simulink model "vehicle_dynamics_blockset_simulation"  (R2020b)
settings: Solver=VariableStepAuto  StartTime=0.0  StopTime=10.0  RelTol=1e-3
values from neighbouring files (symbols this model uses):
  CONST =     [ParamsFull.mat]
  VEHICLE =     [ParamsFull.mat]
undefined symbols (not defined in the file or in its folder): InertFrm, VEH
libraries: sharedtransform x6, sim3dlib x4, vehdynlibtirecommon x4, autolibutils x4, autolibshared x3, vehdynlibtire x2, vehdynlibviscommon x2, vehdynlibsteering x1, simulink x1, sim3dautolib x1
(part 1 of 4)
settings Model: Creator=josip  LastModifiedBy=josip
settings DataIOCC: ReturnWorkspaceOutputs=off
settings DebuggingCC: ArithmeticOperatorsInVariantConditions=warning
settings HardwareCC: ProdBitPerLong=64  ProdHWDeviceType=AMD->x86-64 (Linux 64)
settings SFSimCC: CustomCodeUndefinedFunction=UseInterfaceOnly

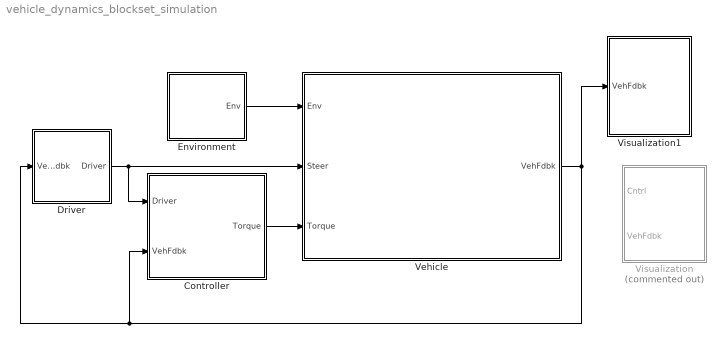
== system vehicle_dynamics_blockset_simulation ==
  Controller : Subsystem
      mask Display: image('images/SystemControllers.png')
  Driver : Subsystem  VariantControl=0
      mask Display: image('images/LongitudinalDriver.png');
  Environment : Subsystem
      mask Display: disp('Environment')
  Vehicle : Subsystem
      mask Display: image('images/PassengerVehicle.png')
  Visualization : Subsystem  Commented=on
      mask Display: disp('Visualization')
  Visualization1 : Subsystem
      mask Display: disp('Visualization')
  wires:
  Environment/1(Env) -> Vehicle/1(Env)
  Driver/1(Driver) -> Controller/1(Driver), Vehicle/2(Steer)
  Vehicle/1(VehFdbk) -> Visualization1/1(VehFdbk), Controller/2(VehFdbk), Driver/1(VehFdbk)
  Controller/1(Torque) -> Vehicle/3(Torque)

== system vehicle_dynamics_blockset_simulation/Controller ==
  Driver : Inport
  VehFdbk : Inport  Port=2
  Constant : Constant  Value=50*ones(4,1)
  Terminator : Terminator
  Terminator1 : Terminator
  Torque : Outport  VectorParamsAs1DForOutWhenUnconnected=off
  wires:
  Driver/1 -> Terminator/1
  VehFdbk/1 -> Terminator1/1
  Constant/1 -> Torque/1

== system vehicle_dynamics_blockset_simulation/Driver ==
  VehFdbk : Inport
  Brake : Constant  Value=0
  Bus Creator1 : BusCreator  Inputs=3
  Bus Selector : BusSelector  Commented=on  OutputSignals=BdyFrm.Cg.Vel.xdot
  Constant : Constant  Commented=on  Value=10
  Dead Zone : DeadZone  Commented=on  LowerValue=-.1  UpperValue=.1  SaturateOnIntegerOverflow=on
  Gas : Constant  Value=0.5
  Ground : Ground  Commented=on
  Longitudinal Driver : autolibshared/Longitudinal Driver  Commented=on  extAccelOvr=off  extDecelOvr=off  extAccelHld=off  extDecelHld=off  extAccelZero=off  extDecelZero=off  cntrlType=PI  shftType=None  velUnits=m/s  gearOut=off  Kp=10  Ki=5  Kff=.1  Kg=0  VehVelVec=[0 100]  KffVec=[.1 .1]  KpVec=[10 10]  KiVec=[5 5]  KgVec=[0 0]  m=1500  Kpt=3000  tau=.1  L=2  aR=200  bR=2.5  cR=.5  g=9.81  vnom=10  Kaw=0  tauerr=0  tauPt=2  GearInit=0  tShift=.1  pdlVec=[0.1 0.4 0.5 0.9]  upShftTbl=[-1 12.9375 26.4375 39.9375 51.18749999999999 62.4375 72.84375 83.25;-1 16.3125 29.8125 43.3125 54.5624 65.8125 76.78125 87.75;-1 19.6875 33.1875 46.68749999999999 57.9375 69.1875 80.71875 92.25;-1 33 52.5 77.25 100.5 138.75 161.875 185]  dwnShftTbl=[1 9.5625 23.0625 36.5625 47.8125 59.0625 68.90625 78.75;1 12.9375 26.4375 39.9375 51.18749999999999 62.4375 72.84375 83.25;1 16.3125 29.8125 43.3125 54.562499 65.8125 76.78125 87.75;1 19.6875 33.1875 46.68749999999999 57.9375 69.1875 80.71875 92.25]  tClutch=.5  tRev=.5  tPark=120  aMode=2  UpGearVec="[0  1  2  3  4  5  6  7]"  DownGearVec="[1  2  3  4  5  6  7  8]"
      settings: SourceProductBaseCode=PW,MT,UV,VE,VP
  Steer : Constant  Value=deg2rad(45)
  Terminator : Terminator
  Terminator1 : Terminator  Commented=on
  Terminator2 : Terminator  Commented=on
  Terminator3 : Terminator  Commented=on
  Driver : Outport  VectorParamsAs1DForOutWhenUnconnected=off
  wires:
  Longitudinal Driver/3 -> Terminator2/1  "Brake"
  Ground/1 -> Longitudinal Driver/3
  Longitudinal Driver/2 -> Terminator1/1  "Accel"
  Bus Creator1/1 -> Driver/1
  Longitudinal Driver/1 -> Terminator3/1
  Bus Selector/1 -> Dead Zone/1  "<xdot>"
  Dead Zone/1 -> Longitudinal Driver/2
  Constant/1 -> Longitudinal Driver/1
  Steer/1 -> Bus Creator1/1  "steer"
  Gas/1 -> Bus Creator1/2  "gas"
  Brake/1 -> Bus Creator1/3  "brake"
  VehFdbk/1 -> Terminator/1

== system vehicle_dynamics_blockset_simulation/Environment ==
  Bus Creator1 : BusCreator  Inputs=2
  Constant3 : Constant  Value=0
  Constant4 : Constant  Value=0
  Constant5 : Constant  Value=0
  Friction : Constant  Value=ones(4,1).*1.0
  Ground Feedback : Subsystem  Variant=on  VariantControlMode=label  LabelModeActiveChoice=0
  Vector Concatenate : Concatenate  NumInputs=3
  Env : Outport  VectorParamsAs1DForOutWhenUnconnected=off
  wires:
  Constant5/1 -> Vector Concatenate/3  "Z"
  Vector Concatenate/1 -> Bus Creator1/1  "Wind"
  Constant3/1 -> Vector Concatenate/1  "X"
  Constant4/1 -> Vector Concatenate/2  "Y"
  Ground Feedback/1(Ground) -> Bus Creator1/2  "Gnd"
  Bus Creator1/1 -> Env/1
  Friction/1 -> Ground Feedback/1(Friction)

== system vehicle_dynamics_blockset_simulation/Vehicle ==
  Env : Inport
  Steer : Inport  Port=2
  Torque : Inport  Port=3
  Bus Selector1 : BusSelector  OutputSignals=Gnd.z.G_FL_z,Gnd.z.G_FR_z,Gnd.z.G_RL_z,Gnd.z.G_RR_z
  Bus Selector2 : BusSelector  OutputSignals=Wind
  Bus Selector3 : BusSelector  OutputSignals=Gnd.mu.mu_FL,Gnd.mu.mu_FR,Gnd.mu.mu_RL,Gnd.mu.mu_RR
  Bus Selector4 : BusSelector  OutputSignals=steer
  Constant : Constant  Value=zeros(4,1)
  PassVeh7DOF : ModelReference  Commented=on  ModelNameDialog=PassVeh7DOF  SimulationMode=Normal  VariantControl=1  ModelReferenceVersion=2.89
  Steering : Subsystem
  Terminator : Terminator
  Vector Concatenate : Concatenate  NumInputs=4
  Vector Concatenate1 : Concatenate  NumInputs=4
  Vehicle : Subsystem
  Wheels and tires : Subsystem  Commented=on
  VehFdbk : Outport  VectorParamsAs1DForOutWhenUnconnected=off
  wires:
  Steer/1 -> Bus Selector4/1
  Steering/1(WhlAng) -> Vehicle/4(WhlAng)
  Torque/1 -> Vehicle/1(AxlTrq)
  Constant/1 -> Vehicle/2(BrkPrs)
  Vehicle/1(Veh) -> VehFdbk/1
  Bus Selector3/1 -> Vector Concatenate/1  "<mu_FL>"
  Bus Selector1/2 -> Vector Concatenate1/2  "<G_FR_z>"
  Vector Concatenate1/1 -> Vehicle/5(Ground)
  Vector Concatenate/1 -> Vehicle/6(Friction)
  Bus Selector1/1 -> Vector Concatenate1/1  "<G_FL_z>"
  Bus Selector3/4 -> Vector Concatenate/4  "<mu_RR>"
  Bus Selector3/2 -> Vector Concatenate/2  "<mu_FR>"
  Bus Selector3/3 -> Vector Concatenate/3  "<mu_RL>"
  Bus Selector1/4 -> Vector Concatenate1/4  "<G_RR_z>"
  Bus Selector1/3 -> Vector Concatenate1/3  "<G_RL_z>"
  Bus Selector2/1 -> Vehicle/3(WindXYZ)  "<Wind>"
  Env/1 -> Bus Selector3/1, Bus Selector1/1, Bus Selector2/1
  Vehicle/2(Wheels) -> Terminator/1
  Bus Selector4/1 -> Steering/1(Steer)  "<steer>"

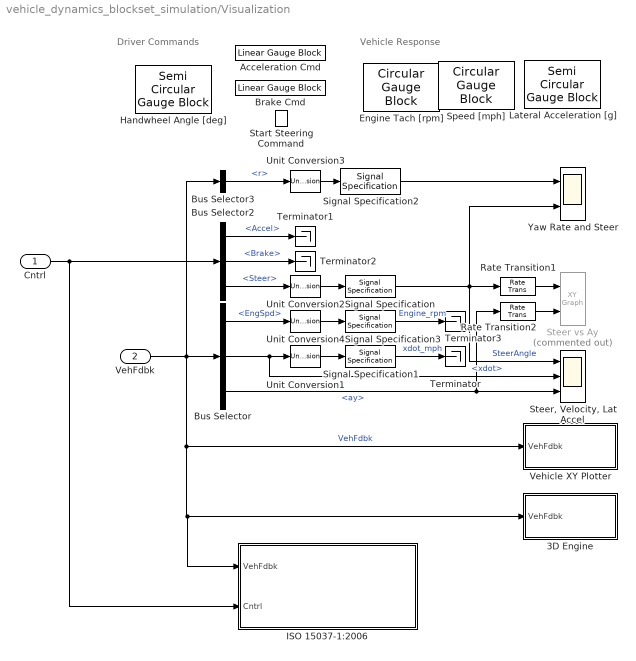
== system vehicle_dynamics_blockset_simulation/Visualization ==
  note: Driver Commands
  note: Vehicle Response
  Cntrl : Inport
  VehFdbk : Inport  Port=2
  3D Engine : Subsystem  Variant=on  VariantControlMode=label  LabelModeActiveChoice=0  mask(3D Engine){engine3D=Disabled, SceneDesc=Open surface, dt3D=.03}
      mask prompts: engine3D "3D Engine"; SceneDesc "Scene Description:"; dt3D "Engine frame rate, dt3D [s]:"
      mask help: This subsystem contains the interface blocks which permit the display of the vehicle in 3D virtual environment. Enable it to view the simulation progress, disable it to inhibit the display.
      mask init:
      | switch get_param(gcb,'engine3D')
      |     case 'Disabled'
      |         set_param(gcb,'OverrideUsingVariant','0')
      |         try
      |             set_param([bdroot '/Environment/Ground Feedback'],'OverrideUsingVariant','0')
      |         catch
      |             disp('No ground feedback sensor found')
      |         end
      |     case 'Enabled'
      |         set_param(gcb,'OverrideUsingVariant','1')
      |         try
      |             set_param([bdroot '/Environment/Ground Feedback'],'OverrideUsingVariant','1')
      |         catch
      |             disp('No ground feedback sensor found')
      |         end
      |     otherwise
      |         set_param(gcb,'OverrideUsingVariant','0')
      | end
      settings: AttributesFormatString=%<engine3D>
      mask Help: eval('vdynblkshelp(''vdynblksscenecameraray'')');
      mask TypeOptions engine3D: Enabled | Disabled
      mask Callback engine3D:
      | switch get_param(gcb,'engine3D')
      |     case 'Disabled'
      |         set_param(gcb,'OverrideUsingVariant','0')
      |     case 'Enabled'
      |        set_param(gcb,'OverrideUsingVariant','1')
      |     otherwise
      |        set_param(gcb,'OverrideUsingVariant','0')
      | end
      mask TypeOptions SceneDesc:
      | 3D Engine/Simulation 3D Engine
      | 1/SceneDesc
      mask Display: disp('3D Engine')
  Acceleration Cmd : LinearGaugeBlock  LabelPosition=Hide  ScaleMax=1  TickInterval=0.20000000000000001
  Brake Cmd : LinearGaugeBlock  LabelPosition=Hide  ScaleMax=1  TickInterval=0.20000000000000001
  Bus Selector : BusSelector  OutputSignals=Driveline.EngSpd,Body.xdot,Body.ay
  Bus Selector2 : BusSelector  OutputSignals=Accel,Brake,Steer
  Bus Selector3 : BusSelector  OutputSignals=Body.r
  Engine Tach [rpm] : CircularGaugeBlock  LabelPosition=Hide  ScaleMax=8000  TickInterval=1000
  Handwheel Angle [deg] : SemiCircularGaugeBlock  LabelPosition=Hide  ScaleMin=-300  ScaleMax=300  TickInterval=60
  ISO 15037-1:2006 : Subsystem  StopFcn=|  Variant=on  VariantControlMode=label  LabelModeActiveChoice=0  mask(ISO 15037-1:2006){Measurement=Disabled}
      | switch get_param(gcb,'Measurement')
      |     case 'Enabled'
      |        p=slproject.getCurrentProject;
      |        projectRoot=p.RootFolder;
      |        SySFolder=fullfile(projectRoot, 'System');
      |        Simulink.sdi.loadView([SySFolder filesep 'ISO15037_1_2006E.mldatx']);
      |        Simulink.sdi.view;
      | end
      mask prompts: Measurement "ISO Measurements"
      mask help: Enables display of ISO 15037-1:2006 standard measurement signals in the Simulation Data Inspector.
      mask init:
      | switch get_param(gcb,'Measurement')
      |     case 'Disabled'
      |         set_param(gcb,'OverrideUsingVariant','0')
      |     case 'Enabled'
      |        set_param(gcb,'OverrideUsingVariant','1')
      |     otherwise
      |        set_param(gcb,'OverrideUsingVariant','0')
      | end
      settings: AttributesFormatString=%<Measurement>
      mask Help: eval('vdynblkshelp(''iso15037'')');
      mask TypeOptions Measurement: Enabled | Disabled
      mask Callback Measurement:
      | switch get_param(gcb,'Measurement')
      |     case 'Disabled'
      |         set_param(gcb,'OverrideUsingVariant','0')
      |     case 'Enabled'
      |        set_param(gcb,'OverrideUsingVariant','1')
      |     otherwise
      |        set_param(gcb,'OverrideUsingVariant','0')
      | end
      mask Display: disp('ISO 15037-1:2006')
  Lateral Acceleration [g] : SemiCircularGaugeBlock  LabelPosition=Hide  ScaleMin=-1  ScaleMax=1  TickInterval=0.5
  Rate Transition1 : RateTransition  Deterministic=off  OutPortSampleTime=.1
  Rate Transition2 : RateTransition  Deterministic=off  OutPortSampleTime=.1
  Signal Specification : SignalSpecification  Unit=deg
  Signal Specification1 : SignalSpecification  Unit=mph
  Signal Specification2 : SignalSpecification  Unit=deg/s
  Signal Specification3 : SignalSpecification  Unit=rpm
  Speed [mph] : CircularGaugeBlock  LabelPosition=Hide  TickInterval=10
  Start Steering Command : LampBlock  LabelPosition=Hide
  Steer vs Ay : simulink/Sinks/XY Graph  Commented=on  xmin=-300  xmax=300  ymin=-1.5  ymax=1.5  st=.1
  "Steer, Velocity, Lat Accel" : Scope  NumInputPorts=3
  Terminator{,1..3} (4 alike) : Terminator
  Unit Conversion{1..4} (4 alike) : UnitConversion
  Vehicle XY Plotter : Subsystem  mask(Vehicle XY Plotter){a=VEHICLE.LF, b=VEHICLE.LR, w=VEHICLE.TRACK_FRONT, figBorder=30, bufferSize=1024, pltDT=.1}
      mask prompts: a "Distance to front axle from CG, a [m]:"; b "Distance to rear axle from CG, b [m]:"; w "Track width, w [m]:"; figBorder "Distance to figure borders, figBorder [m]:"; bufferSize "Path buffer sampe size, bufferSize []:"; pltDT "Plot update rate, pltDT [s]:"
      mask help: This block will display a MATLAB figure which indicates the vehicle path, current position and heading velocity.
      mask TypeOptions a: Vehicle XY Plotter/a
      mask TypeOptions b: Vehicle XY Plotter/b
      mask TypeOptions w: Vehicle XY Plotter/w
      mask TypeOptions figBorder: Vehicle XY Plotter/figBorder
      mask TypeOptions bufferSize: Vehicle XY Plotter/bufferSize
  Yaw Rate and Steer : Scope  NumInputPorts=2
  wires:
  Unit Conversion3/1 -> Signal Specification2/1
  Bus Selector3/1 -> Unit Conversion3/1  "<r>"
  Signal Specification2/1 -> Yaw Rate and Steer/1
  Unit Conversion4/1 -> Signal Specification3/1
  Signal Specification3/1 -> Terminator3/1  "Engine_rpm"
  Signal Specification/1 -> Yaw Rate and Steer/2, Rate Transition1/1, "Steer, Velocity, Lat Accel"/1  "SteerAngle"
  Bus Selector2/3 -> Unit Conversion2/1  "<Steer>"
  Signal Specification1/1 -> Terminator/1  "xdot_mph"
  Unit Conversion1/1 -> Signal Specification1/1
  Bus Selector/3 -> Rate Transition2/1, "Steer, Velocity, Lat Accel"/3  "<ay>"
  Bus Selector2/1 -> Terminator1/1  "<Accel>"
  Rate Transition1/1 -> Steer vs Ay/1
  Unit Conversion2/1 -> Signal Specification/1
  Bus Selector/2 -> "Steer, Velocity, Lat Accel"/2, Unit Conversion1/1  "<xdot>"
  VehFdbk/1 -> Bus Selector3/1, Bus Selector/1, Vehicle XY Plotter/1(VehFdbk), 3D Engine/1(VehFdbk), ISO 15037-1:2006/1(VehFdbk)  "VehFdbk"
  Cntrl/1 -> ISO 15037-1:2006/2(Cntrl), Bus Selector2/1
  Rate Transition2/1 -> Steer vs Ay/2
  Bus Selector/1 -> Unit Conversion4/1  "<EngSpd>"
  Bus Selector2/2 -> Terminator2/1  "<Brake>"

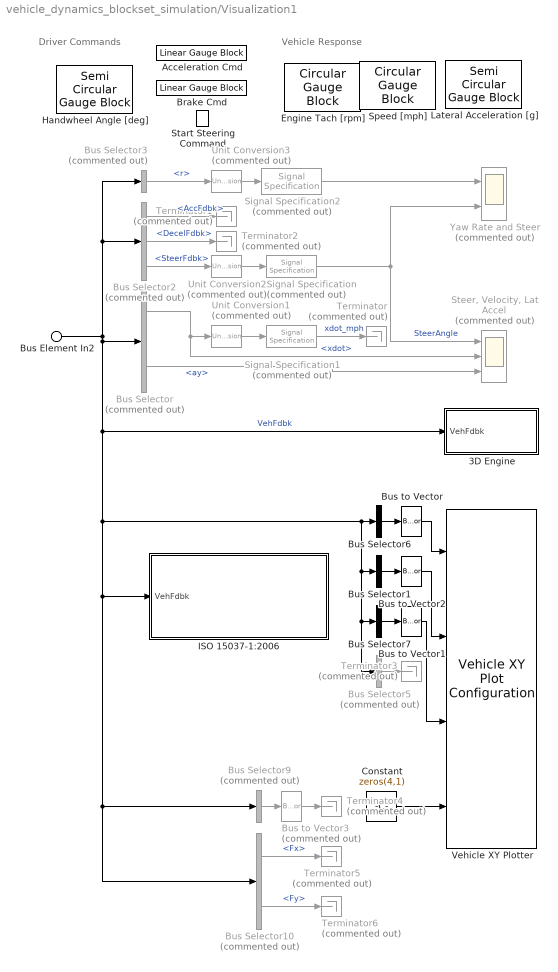
== system vehicle_dynamics_blockset_simulation/Visualization1 ==
  note: Driver Commands
  note: Vehicle Response
  Bus Element In2 : Inport  PortName=VehFdbk
  3D Engine : Subsystem  Variant=on  VariantControlMode=label  LabelModeActiveChoice=0  mask(3D Engine){engine3D=Disabled, SceneDesc=Open surface, dt3D=.03, defaultPos=Recommended for scene, X_o=0, Y_o=0, Z_o=0, phi_o=0, theta_o=0, psi_o=0}
      mask prompts: engine3D "3D Engine"; SceneDesc "Scene:"; dt3D "Engine frame rate, dt3D [s]:"; X_o "Initial longitudinal position, X_o [m]:"; Y_o "Initial lateral position, Y_o [m]:"; Z_o "Initial vertical position, Z_o [m]:"; phi_o "Initial roll angle, phi_o [rad]:"; theta_o "Initial pitch angle, theta_o [rad]:"; psi_o "Initial yaw angle, psi_o [rad]:"
      mask help: This subsystem contains the interface blocks which permit the display of the vehicle in the 3D virtual environment. Enable it to view the simulation progress, disable it to inhibit the display.
      mask init:
      | switch get_param(gcb,'engine3D')
      |     case 'Disabled'
      |         set_param(gcb,'OverrideUsingVariant','0')
      |         try
      |             set_param([bdroot '/Environment/Ground Feedback'],'OverrideUsingVariant','0')
      |         catch
      |             disp('Warning: No ground feedback sensor not set')
      |         end
      |     case 'Enabled'
      |         set_param(gcb,'OverrideUsingVariant','1')
      |         try
      |             set_param([bdroot '/Environment/Ground Feedback'],'OverrideUsingVariant','1')
      |         catch
      |             disp('Warning: No ground feedback sensor not set')
      |         end
      |     otherwise
      |         set_param(gcb,'OverrideUsingVariant','0')
      | end
      settings: AttributesFormatString=|
      | %<SceneDesc>
      | %<engine3D>
      mask Help: eval('vdynblkshelp(''vdynblks3dengine'')');
      mask TypeOptions engine3D: Enabled | Disabled
      mask Callback engine3D:
      | switch get_param(gcb,'engine3D')
      |     case 'Disabled'
      |         set_param(gcb,'OverrideUsingVariant','0')
      |     case 'Enabled'
      |        set_param(gcb,'OverrideUsingVariant','1')
      |     otherwise
      |        set_param(gcb,'OverrideUsingVariant','0')
      | end
      mask TypeOptions SceneDesc: 3D Engine/Simulation 3D Scene Configuration/SceneDesc
      mask Callback SceneDesc:
      | defaultStatus = get_param(gcb,'defaultPos');
      | if strcmp(defaultStatus,'Recommended for scene')
      | sceneType = get_param(gcb,'SceneDesc');
      | switch sceneType
      |     case 'Straight road'
      |         set_param(gcb,'X_o', '-118')
      |         set_param(gcb,'Y_o', '3.125')
      |         set_param(gcb,'Z_o', '0')
      |         set_param(gcb,'phi_o', '0')
      |         set_param(gcb,'theta_o', '0')
      |         set_param(gcb,'psi_o', '0')
      |     case 'Curved road'
      |         set_param(gcb,'X_o', '0.2')
      |         set_param(gcb,'Y_o', '-1605.0')
      |         set_param(gcb,'Z_o', '0')
      |         set_param(gcb,'phi_o', '0')
      |         set_param(gcb,'theta_o', '0')
      |         set_param(gcb,'psi_o', '-156*pi/180')
      |     case 'Parking lot'
      |         set_param(gcb,'X_o', '-104.0')
      |         set_param(gcb,'Y_o', '-9.7')
      |         set_param(gcb,'Z_o', '0')
      |         set_param(gcb,'phi_o', '0')
      |         set_param(gcb,'theta_o', '0')
      |         set_param(gcb,'psi_o', '0')
      |     case 'Double lane change'
      |         set_param(gcb,'X_o', '0')
      |         set_param(gcb,'Y_o', '3.125')
      |         set_param(gcb,'Z_o', '0')
      |         set_param(gcb,'phi_o', '0')
      |         set_param(gcb,'theta_o', '0')
      |         set_param(gcb,'psi_o', '0')
      |     case 'Open surface'
      |         set_param(gcb,'X_o', '0')
      |         set_param(gcb,'Y_o', '0')
      |         set_param(gcb,'Z_o', '0')
      |         set_param(gcb,'phi_o', '0')
      |         set_param(gcb,'theta_o', '0')
      |         set_param(gcb,'psi_o', '0')
      |     case 'US highway'
      |         set_param(gcb,'X_o', '3592.00')
      |         set_param(gcb,'Y_o', '2617.00')
      |         set_param(gcb,'Z_o', '-1.0')
      |         set_param(gcb,'phi_o', '0')
      |         set_param(gcb,'theta_o', '0')
      |         set_param(gcb,'psi_o', '0')
      |     case 'US city block'
      |         set_param(gcb,'X_o', '-125.19')
      |         set_param(gcb,'Y_o', '1.65')
      |         set_param(gcb,'Z_o', '-0.04')
      |         set_param(gcb,'phi_o', '0')
      |         set_param(gcb,'theta_o', '0')
      |         set_param(gcb,'psi_o', '0')
      |     case 'Large parking lot'
      |         set_param(gcb,'X_o', '45.0')
      |         set_param(gcb,'Y_o', '54.7')
      |         set_param(gcb,'Z_o', '0.0')
      |         set_param(gcb,'phi_o', '0')
      |         set_param(gcb,'theta_o', '0')
      |         set_param(gcb,'psi_o', '-pi/2')
      |     case 'Virtual Mcity'
      |         set_param(gcb,'X_o', '-26.0')
      |         set_param(gcb,'Y_o', '76.0')
      |         set_param(gcb,'Z_o', '0.0')
      |         set_param(gcb,'phi_o', '0')
      |         set_param(gcb,'theta_o', '0')
      |         set_param(gcb,'psi_o', '-40*pi/180')
      |     otherwise
      |         set_param(gcb,'X_o', '0')
      |         set_param(gcb,'Y_o', '0')
      |         set_param(gcb,'Z_o', '0')
      |         set_param(gcb,'phi_o', '0')
      |         set_param(gcb,'theta_o', '0')
      |         set_param(gcb,'psi_o', '0')
      | end
      | end
      mask TypeOptions defaultPos: Recommended for scene | User-specified
      mask DialogControl engineConfig Prompt: 3D Engine Settings
      mask DialogControl posSetup Prompt: Initial vehicle position
      mask DialogControl posSetupDesc Prompt: To use these initial vehicle positions, first Apply the initial values and then click Update the model workspaces with the initial values.
      mask DialogControl setModelPos Prompt: Update model workspaces with initial values
      mask DialogControl setModelPos Callback:
      | if strcmp(get_param(bdroot(gcb),'SimulationStatus'),'stopped')
      |     aMaskObj = Simulink.Mask.get(gcbh);
      |     aDlgHdl = aMaskObj.getDialogHandle();
      |     if ~isempty(aDlgHdl)
      |         aDlgHdl.apply;
      |     end
      |     sceneType = get_param(gcb,'SceneDesc');
      |     rootModel = bdroot(gcb);
      |     ws = get_param(rootModel, 'modelworkspace');
      |     VEH = getVariable(ws,'VEH');
      |     ParamList={'X_o',[1,1],{};'Y_o',[1,1],{};'Z_o',[1,1],{};'phi_o',[1,1],{'gte',-pi/2;'lte',pi/2};'theta_o',[1,1],{'gte',-pi/2;'lte',pi/2};'psi_o',[1,1],{'gte',-2*pi;'lte',2*pi}};
      |     paramStruct = autoblkscheckparams(gcb, '3D Engine',ParamList);
      |     VEH.InitialLongPosition = paramStruct.X_o;
      |     VEH.InitialLatPosition = paramStruct.Y_o;
      |     VEH.InitialVertPosition = paramStruct.Z_o;
      |     VEH.InitialRollAngle = paramStruct.phi_o;
      |     VEH.InitialPitchAngle = paramStruct.theta_o;
      |     VEH.InitialYawAngle = paramStruct.psi_o;
      |     assignin(ws,'VEH',VEH);
      |     modelList = {'PassVeh14DOF','PassVeh7DOF'};
      |     for idx =1:length(modelList)
      | %         try
      |             load_system(modelList{idx});
      |             ws = get_param(modelList{idx}, 'modelworkspace');
      |             assignin(ws,'VEH',VEH);
      |             save_system(modelList{idx});
      |             close_system(modelList{idx});
      | %         catch
      | %             disp(['Cannot find ' modelList{idx}])
      | %         end
      |     end
      | end
      mask Display: disp('3D Engine')
  Acceleration Cmd : LinearGaugeBlock  LabelPosition=Hide  ScaleMax=1  TickInterval=0.20000000000000001
  Brake Cmd : LinearGaugeBlock  LabelPosition=Hide  ScaleMax=1  TickInterval=0.20000000000000001
  Bus Selector : BusSelector  Commented=on  OutputSignals=BdyFrm.Cg.Vel.xdot,BdyFrm.Cg.Acc.ay
  Bus Selector1 : BusSelector  OutputSignals=InertFrm.Cg.Ang.phi,InertFrm.Cg.Ang.theta,InertFrm.Cg.Ang.psi  OutputAsBus=on
  Bus Selector10 : BusSelector  Commented=on  OutputSignals=Wheels.TireFrame.Fx,Wheels.TireFrame.Fy
  Bus Selector2 : BusSelector  Commented=on  OutputSignals=Driver.AccFdbk,Driver.DecelFdbk,Driver.SteerFdbk
  Bus Selector3 : BusSelector  Commented=on  OutputSignals=Body.BdyFrm.Cg.AngVel.r
  Bus Selector5 : BusSelector  Commented=on  OutputSignals=Driveline.WhlAng  OutputAsBus=on
  Bus Selector6 : BusSelector  OutputSignals=InertFrm.Geom.Disp.X,InertFrm.Geom.Disp.Y,InertFrm.Geom.Disp.Z  OutputAsBus=on
  Bus Selector7 : BusSelector  OutputSignals=InertFrm.Cg.Vel.Xdot,InertFrm.Cg.Vel.Ydot,InertFrm.Cg.Vel.Zdot  OutputAsBus=on
  Bus Selector9 : BusSelector  Commented=on  OutputSignals=Driveline.EngSpd,Driveline.Gear  OutputAsBus=on
  Bus to Vector : BusToVector
  Bus to Vector1 : BusToVector
  Bus to Vector2 : BusToVector
  Bus to Vector3 : BusToVector  Commented=on
  Constant : Constant  Value=zeros(4,1)
  Engine Tach [rpm] : CircularGaugeBlock  LabelPosition=Hide  ScaleMax=8000  TickInterval=1000
  Handwheel Angle [deg] : SemiCircularGaugeBlock  LabelPosition=Hide  ScaleMin=-300  ScaleMax=300  TickInterval=60
  ISO 15037-1:2006 : Subsystem  StopFcn=|  Variant=on  VariantControlMode=label  LabelModeActiveChoice=0  mask(ISO 15037-1:2006){Measurement=Disabled}
      | switch get_param(gcb,'Measurement')
      |     case 'Enabled'
      |        p=slproject.getCurrentProject;
      |        projectRoot=p.RootFolder;
      |        SySFolder=fullfile(projectRoot, 'System');
      |        Simulink.sdi.loadView([SySFolder filesep 'ISO15037_1_2006E.mldatx']);
      |        Simulink.sdi.view;
      | end
      mask prompts: Measurement "ISO Measurements"
      mask help: Enables display of ISO 15037-1:2006 standard measurement signals in the Simulation Data Inspector.
      mask init: same as vehicle_dynamics_blockset_simulation/Visualization/ISO 15037-1:2006
      settings: AttributesFormatString=%<Measurement>
      mask Help: eval('vdynblkshelp(''iso15037'')');
      mask TypeOptions Measurement: Enabled | Disabled
      mask Callback Measurement:
      | switch get_param(gcb,'Measurement')
      |     case 'Disabled'
      |         set_param(gcb,'OverrideUsingVariant','0')
      |     case 'Enabled'
      |        set_param(gcb,'OverrideUsingVariant','1')
      |     otherwise
      |        set_param(gcb,'OverrideUsingVariant','0')
      | end
      mask Display: disp('ISO 15037-1:2006')
  Lateral Acceleration [g] : SemiCircularGaugeBlock  LabelPosition=Hide  ScaleMin=-1  ScaleMax=1  TickInterval=0.5
  Signal Specification : SignalSpecification  Commented=on  Unit=deg
  Signal Specification1 : SignalSpecification  Commented=on  Unit=mph
  Signal Specification2 : SignalSpecification  Commented=on  Unit=deg/s
  Speed [mph] : CircularGaugeBlock  LabelPosition=Hide  TickInterval=10
  Start Steering Command : LampBlock  LabelPosition=Hide
  "Steer, Velocity, Lat Accel" : Scope  Commented=on  NumInputPorts=3
  Terminator{,1..6} (7 alike) : Terminator  Commented=on
  Unit Conversion1 : UnitConversion  Commented=on
  Unit Conversion2 : UnitConversion  Commented=on
  Unit Conversion3 : UnitConversion  Commented=on
  Vehicle XY Plotter : vehdynlibviscommon/Vehicle XY Plot Configuration  extRef=off  extStats=off  extTireF=off  a=VEHICLE.LF  b=VEHICLE.LR  w=VEHICLE.TRACK_FRONT  figBorder=10  bufferSize=1024  velNorm=5  tireFNorm=1000  pltDT=.1
      settings: SourceProductBaseCode=VE
  Yaw Rate and Steer : Scope  Commented=on  NumInputPorts=2
  wires:
  Unit Conversion3/1 -> Signal Specification2/1
  Bus Selector3/1 -> Unit Conversion3/1  "<r>"
  Signal Specification2/1 -> Yaw Rate and Steer/1
  Bus Selector/2 -> "Steer, Velocity, Lat Accel"/3  "<ay>"
  Bus Element In2/1 -> Bus Selector10/1, Bus Selector9/1, ISO 15037-1:2006/1(VehFdbk), Bus Selector5/1, Bus Selector7/1, Bus Selector1/1, Bus Selector6/1, 3D Engine/1(VehFdbk), Bus Selector/1, Bus Selector3/1, Bus Selector2/1  "VehFdbk"
  Bus Selector2/2 -> Terminator2/1  "<DecelFdbk>"
  Bus to Vector2/1 -> Vehicle XY Plotter/2
  Bus Selector6/1 -> Bus to Vector/1
  Bus to Vector/1 -> Vehicle XY Plotter/1
  Bus Selector1/1 -> Bus to Vector2/1
  Bus to Vector1/1 -> Vehicle XY Plotter/3
  Bus Selector7/1 -> Bus to Vector1/1
  Bus Selector2/1 -> Terminator1/1  "<AccFdbk>"
  Bus Selector2/3 -> Unit Conversion2/1  "<SteerFdbk>"
  Bus Selector10/2 -> Terminator6/1  "<Fy>"
  Signal Specification1/1 -> Terminator/1  "xdot_mph"
  Unit Conversion1/1 -> Signal Specification1/1
  Signal Specification/1 -> Yaw Rate and Steer/2, "Steer, Velocity, Lat Accel"/1  "SteerAngle"
  Bus Selector10/1 -> Terminator5/1  "<Fx>"
  Unit Conversion2/1 -> Signal Specification/1
  Bus Selector/1 -> "Steer, Velocity, Lat Accel"/2, Unit Conversion1/1  "<xdot>"
  Bus Selector5/1 -> Terminator3/1
  Constant/1 -> Vehicle XY Plotter/4
  Bus to Vector3/1 -> Terminator4/1
  Bus Selector9/1 -> Bus to Vector3/1

== system vehicle_dynamics_blockset_simulation/Environment/Ground Feedback ==
  note: 1) Add Subsystem or Model blocks as valid variant choices.
      | 2) You cannot connect blocks at this level. At simulation, connectivity is automatically
      | determined, based on the active variant and port name matching.
  Friction : Inport
  3D Engine : Subsystem  VariantControl=1
  Constant : Subsystem  VariantControl=0
  Ground : Outport  VectorParamsAs1DForOutWhenUnconnected=off

== system vehicle_dynamics_blockset_simulation/Vehicle/Steering ==
  Steer : Inport
  Constant : Constant  Value=0
  Kinematic Steering : vehdynlibsteering/Kinematic Steering  StrgType=Parallel  StrgRatioType=Constant  Loc=Front  NrmlFctr=0.01  TrckWdth=1  WhlBase=1.524  Db=0  StrgRng=VEHICLE.MAX_STEERING_ANGLE/VEHICLE.STEERING_RATIO  StrgAngBpts="[-6.2832   -5.0265   -3.7699   -2.5133   -1.2566         0    1.2566    2.5133    3.7699    5.0265    6.2832]"  StrgRatioTbl=|  StrgRatio=VEHICLE.STEERING_RATIO  StrgArmLngth=0.1  RckCsLngth=0.5  TieRodLngth=0.248  D=0.2  PnnRadius=0.0057  PnnRadiusTbl="[0.0055    0.0055    0.0056    0.0057    0.0058    0.0057    0.0057    0.0057    0.0056    0.0055    0.0055]"  RodLngth=0.1  ParaArmLngth=0.9  aMode=2
      | [13.5000   13.3750   13.2500   13.1250   13.0000   13.0000   13.0000   13.1250   13.2500   13.3750   13.5000
      | ]
  Terminator : Terminator
  Vector Concatenate : Concatenate
  Vector Concatenate1 : Concatenate
  Vector Concatenate2 : Concatenate
  WhlAng : Outport  Unit=rad  VectorParamsAs1DForOutWhenUnconnected=off
  wires:
  Kinematic Steering/1 -> Terminator/1
  Steer/1 -> Kinematic Steering/1
  Kinematic Steering/2 -> Vector Concatenate/1
  Vector Concatenate2/1 -> Vector Concatenate1/2  "RearWheelAngles"
  Vector Concatenate/1 -> Vector Concatenate1/1  "FrontWheelAngles"
  Vector Concatenate1/1 -> WhlAng/1
  Kinematic Steering/3 -> Vector Concatenate/2
  Constant/1 -> Vector Concatenate2/2, Vector Concatenate2/1

== system vehicle_dynamics_blockset_simulation/Vehicle/Vehicle ==
  AxlTrq : Inport  Unit=N*m  PortDimensions=4
  BrkPrs : Inport  Port=2  Unit=Pa  PortDimensions=4
  WindXYZ : Inport  Port=3  PortDimensions=3
  WhlAng : Inport  Port=4  Unit=rad  PortDimensions=4
  Ground : Inport  Port=5  Unit=m  PortDimensions=4
  Friction : Inport  Port=6  Unit=1  PortDimensions=4
  Bus Selector : BusSelector  OutputSignals=InertFrm,BdyFrm  OutputAsBus=on
  Longitudinal Wheels 4DOF : Subsystem  VariantControl=1
      settings: AttributesFormatString=%<wheelMode>
  Vehicle Body 3DOF External Longitudinal Wheels : Subsystem  Variant=on  VariantControlMode=label  VariantControl=Variant1  LabelModeActiveChoice=1
      settings: AttributesFormatString=%<trackMode>
  Vehicle Signal Routing : Subsystem
  Bus Element Out3 : Outport  PortName=Veh
  Bus Element Out1 : Outport  Port=2  PortName=Wheels
  wires:
  Longitudinal Wheels 4DOF/3(Wheels) -> Bus Element Out1/1  "Wheels"
  WhlAng/1 -> Vehicle Body 3DOF External Longitudinal Wheels/1(WhlAng), Longitudinal Wheels 4DOF/1(WhlAng)
  Bus Selector/1 -> Bus Element Out3/1
  Friction/1 -> Longitudinal Wheels 4DOF/4(Friction)
  Vehicle Signal Routing/1(Veh) -> Bus Selector/1
  Longitudinal Wheels 4DOF/2(RearAxlF) -> Vehicle Body 3DOF External Longitudinal Wheels/3("FwR ")
  Vehicle Body 3DOF External Longitudinal Wheels/1(" Info") -> Vehicle Signal Routing/1(Info), Longitudinal Wheels 4DOF/6(VehFdbk)
  WindXYZ/1 -> Vehicle Body 3DOF External Longitudinal Wheels/4(WindXYZ)
  Longitudinal Wheels 4DOF/1(FrntAxlF) -> Vehicle Body 3DOF External Longitudinal Wheels/2("FwF ")
  Ground/1 -> Vehicle Signal Routing/2(Ground), Longitudinal Wheels 4DOF/5(Ground)
  BrkPrs/1 -> Longitudinal Wheels 4DOF/3(BrkPrs)
  AxlTrq/1 -> Longitudinal Wheels 4DOF/2(AxlTrq)

== system vehicle_dynamics_blockset_simulation/Vehicle/Wheels and tires ==
  WheelAng : Inport
  AxleTrq : Inport  Port=2
  BrkPrs : Inport  Port=3
  VehFdbk : Inport  Port=4
  Axle Forces : Subsystem  Commented=on  Variant=on  VariantControlMode=label  LabelModeActiveChoice=1
  Bus Selector5 : BusSelector  OutputSignals=BdyFrm.Cg.AngVel.r
  Constant : vehdynlibtirecommon/Constant  const=220000  numWheels=4
      settings: SourceProductBaseCode=VE
  Constant3 : vehdynlibtirecommon/Constant  const=0  numWheels=4
      settings: SourceProductBaseCode=VE
  Terminator2 : Terminator
  Tire2Veh : Subsystem
  Tires : Subsystem
  Veh2Tire : Subsystem
  Velocity and Vertical Load : Subsystem  Variant=on  VariantControlMode=label  LabelModeActiveChoice=1
  Wheel Angles : Subsystem
  FrntAxlF : Outport  Unit=N  VectorParamsAs1DForOutWhenUnconnected=off
  RearAxlF : Outport  Port=2  Unit=N  VectorParamsAs1DForOutWhenUnconnected=off
  omega : Outport  Port=3  VectorParamsAs1DForOutWhenUnconnected=off
  wires:
  Veh2Tire/4(ydotAxle) -> Tires/4(Vy)  "Vy"
  Veh2Tire/1(T) -> Tires/1(DriveTorque)
  Velocity and Vertical Load/2(Fz) -> Tires/8(Fz)
  Tires/1(Wheels) -> Tire2Veh/1(Wheels)
  Bus Selector5/1 -> Veh2Tire/3(r)  "<r>"
  Veh2Tire/2(P) -> Tires/2(Brake Pressure)
  Velocity and Vertical Load/1(VehV) -> Veh2Tire/4(VehVel)
  Tire2Veh/1(FwF) -> FrntAxlF/1
  Wheel Angles/1(Vehicle) -> Veh2Tire/5(WheelSteer)
  WheelAng/1 -> Wheel Angles/1(WheelAng)  "FrontWheelAngles"
  VehFdbk/1 -> Bus Selector5/1, Velocity and Vertical Load/1(VehFdbk)
  AxleTrq/1 -> Veh2Tire/1(Axle)
  Veh2Tire/3(xdotAxle) -> Tires/3(Vx)  "Vx"
  Veh2Tire/6(zdotAxle) -> Terminator2/1
  BrkPrs/1 -> Veh2Tire/2(Brake)
  Tire2Veh/2(FwR) -> RearAxlF/1
  Constant3/1 -> Wheel Angles/2(Camber), Tires/6(Camber)
  Tire2Veh/3(omega) -> omega/1
  Constant/1 -> Tires/7(Press)
  Veh2Tire/5(psidot) -> Tires/5(r)

== system vehicle_dynamics_blockset_simulation/Visualization/3D Engine ==
  note: 1) Add Subsystem or Model blocks as valid variant choices.
      | 2) You cannot connect blocks at this level. At simulation, connectivity is automatically
      | determined, based on the active variant and port name matching.
  VehFdbk : Inport
  3D Engine : Subsystem  VariantControl=1
  3D Engine Disabled : Subsystem  VariantControl=0

== system vehicle_dynamics_blockset_simulation/Visualization/ISO 15037-1:2006 ==
  VehFdbk : Inport
  Cntrl : Inport  Port=2
  Disabled : Subsystem  VariantControl=0
  Enabled : Subsystem  VariantControl=1

== system vehicle_dynamics_blockset_simulation/Visualization/Vehicle XY Plotter ==
  VehFdbk : Inport
  Bus Selector1 : BusSelector  OutputSignals=Body.phi,Body.theta,Body.psi  OutputAsBus=on
  Bus Selector2 : BusSelector  OutputSignals=Driveline.WhlAng  OutputAsBus=on
  Bus Selector3 : BusSelector  OutputSignals=Body.GeomX,Body.GeomY,Body.GeomZ  OutputAsBus=on
  Bus Selector4 : BusSelector  OutputSignals=Body.GeomXdot,Body.GeomYdot,Body.GeomZdot  OutputAsBus=on
  Bus to Vector{,1..3} (4 alike) : BusToVector
  Rate Transition5 : RateTransition  Deterministic=off  OutPortSampleTime=pltDT
  Vehicle XY Plotter : vehdynlibviscommon/Vehicle XY Plotter  w=w  a=a  b=b  figBorder=figBorder  bufferSize=bufferSize  extStats=off  extTireF=off
      settings: SourceProductBaseCode=VE
  wires:
  Bus to Vector2/1 -> Vehicle XY Plotter/2  "InertCGDisp"
  Bus Selector4/1 -> Bus to Vector1/1
  Bus to Vector1/1 -> Vehicle XY Plotter/3  "InertCGVel"
  Bus Selector1/1 -> Bus to Vector2/1
  Bus to Vector/1 -> Vehicle XY Plotter/1  "InertCGDisp"
  Bus Selector3/1 -> Bus to Vector/1
  Bus Selector2/1 -> Bus to Vector3/1
  VehFdbk/1 -> Rate Transition5/1
  Bus to Vector3/1 -> Vehicle XY Plotter/4  "delta"
  Rate Transition5/1 -> Bus Selector1/1, Bus Selector2/1, Bus Selector4/1, Bus Selector3/1

== system vehicle_dynamics_blockset_simulation/Visualization1/3D Engine ==
  note: 1) Add Subsystem or Model blocks as valid variant choices.
      | 2) You cannot connect blocks at this level. At simulation, connectivity is automatically
      | determined, based on the active variant and port name matching.
  VehFdbk : Inport
  3D Engine : Subsystem  VariantControl=1
  3D Engine Disabled : Subsystem  VariantControl=0

== system vehicle_dynamics_blockset_simulation/Visualization1/ISO 15037-1:2006 ==
  VehFdbk : Inport
  Disabled : Subsystem  VariantControl=0
  Enabled : Subsystem  VariantControl=1

== system vehicle_dynamics_blockset_simulation/Environment/Ground Feedback/3D Engine ==
  Friction : Inport
  Bus Creator : BusCreator  Inputs=4
  Bus Creator2 : BusCreator  Inputs=4
  Bus Creator3 : BusCreator  Inputs=2
  Bus Selector : BusSelector  OutputSignals=HitLoc
  Data Type Conversion : DataTypeConversion
  Demux : Demux
  Demux1 : Demux
  Passenger Vehicle Ray Trace Set : sim3dlib/Vehicle Terrain Sensor  ActorTag=SimulinkVehicle1  VehExtEn=Constant  TireRadiiExt=Constant  VehCntrLngthVal=0  TireRadiiVal=0  VehRayLngth=10  LfRayLngth=20  RfRayLngth=20  LrRayLngth=20  RrRayLngth=20  VehRayOffset=0  LfRayOffset=-1  RfRayOffset=-1  LrRayOffset=-1  RrRayOffset=-1  VehEn=on  LfEn=on  RfEn=on  LrEn=on  RrEn=on  DbgEn=off  Ts=.03  aMode=aMode
      settings: SourceProductBaseCode=DR,UV,VE
  Rate Transition : RateTransition
  Reshape10 : Reshape  OutputDimensionality=Row vector (2-D)
  Selector1 : Selector  InputPortWidth=5  IndexOptions=Index vector (dialog)  Indices=[2:5]  OutputSizes=1
  Signal Specification : SignalSpecification  Unit=m
  Signal Specification1 : SignalSpecification  Unit=1
  Terminator1 : Terminator
  Terminator2 : Terminator
  Zend Select : Selector  NumberOfDimensions=2  InputPortWidth=3  IndexOptions=Select all,Index vector (dialog)  Indices=[1 3],3  OutputSizes=1,1
  Ground : Outport  VectorParamsAs1DForOutWhenUnconnected=off
  wires:
  Selector1/1 -> Rate Transition/1
  Zend Select/1 -> Reshape10/1
  Bus Selector/1 -> Zend Select/1  "<HitLoc>"
  Passenger Vehicle Ray Trace Set/2 -> Terminator1/1
  Passenger Vehicle Ray Trace Set/3 -> Terminator2/1
  Reshape10/1 -> Selector1/1
  Passenger Vehicle Ray Trace Set/1 -> Bus Selector/1
  Rate Transition/1 -> Data Type Conversion/1
  Demux/2 -> Bus Creator/2  "G_FR_z"
  Demux/1 -> Bus Creator/1  "G_FL_z"
  Demux/4 -> Bus Creator/4  "G_RR_z"
  Demux/3 -> Bus Creator/3  "G_RL_z"
  Signal Specification/1 -> Demux/1
  Signal Specification1/1 -> Demux1/1
  Demux1/1 -> Bus Creator2/1  "mu_FL"
  Bus Creator/1 -> Bus Creator3/1  "z"
  Demux1/3 -> Bus Creator2/3  "mu_RL"
  Demux1/4 -> Bus Creator2/4  "mu_RR"
  Demux1/2 -> Bus Creator2/2  "mu_FR"
  Bus Creator2/1 -> Bus Creator3/2  "mu"
  Bus Creator3/1 -> Ground/1
  Friction/1 -> Signal Specification1/1
  Data Type Conversion/1 -> Signal Specification/1

== system vehicle_dynamics_blockset_simulation/Environment/Ground Feedback/Constant ==
  Friction : Inport
  Bus Creator : BusCreator  Inputs=4
  Bus Creator2 : BusCreator  Inputs=4
  Bus Creator3 : BusCreator  Inputs=2
  Constant1 : Constant  Value=zeros(4,1)
  Demux : Demux
  Demux1 : Demux
  Signal Specification : SignalSpecification  Unit=m
  Signal Specification1 : SignalSpecification  Unit=1
  Ground : Outport  VectorParamsAs1DForOutWhenUnconnected=off
  wires:
  Constant1/1 -> Signal Specification/1
  Signal Specification/1 -> Demux/1
  Demux/4 -> Bus Creator/4  "G_RR_z"
  Demux/1 -> Bus Creator/1  "G_FL_z"
  Demux/3 -> Bus Creator/3  "G_RL_z"
  Demux/2 -> Bus Creator/2  "G_FR_z"
  Bus Creator/1 -> Bus Creator3/1  "z"
  Demux1/3 -> Bus Creator2/3  "mu_RL"
  Demux1/4 -> Bus Creator2/4  "mu_RR"
  Demux1/1 -> Bus Creator2/1  "mu_FL"
  Demux1/2 -> Bus Creator2/2  "mu_FR"
  Bus Creator2/1 -> Bus Creator3/2  "mu"
  Friction/1 -> Signal Specification1/1
  Signal Specification1/1 -> Demux1/1
  Bus Creator3/1 -> Ground/1

== system vehicle_dynamics_blockset_simulation/Vehicle/Vehicle/Longitudinal Wheels 4DOF ==
  WhlAng : Inport
  AxlTrq : Inport  Port=2
  BrkPrs : Inport  Port=3
  Friction : Inport  Port=4  PortDimensions=4
  Ground : Inport  Port=5  PortDimensions=4
  VehFdbk : Inport  Port=6
  Axle Forces : Subsystem  Variant=on  VariantControlMode=label  LabelModeActiveChoice=1
  Bus Selector5 : BusSelector  OutputSignals=BdyFrm.Cg.AngVel.r
  Constant : vehdynlibtirecommon/Constant  const=220000  numWheels=4
      settings: SourceProductBaseCode=VE
  Constant3 : vehdynlibtirecommon/Constant  const=0  numWheels=4
      settings: SourceProductBaseCode=VE
  Terminator2 : Terminator
  Tires : Subsystem  Variant=on  VariantControlMode=label  VariantControl=Choice  LabelModeActiveChoice=0
  Veh2Tire : Subsystem
  Velocity and Vertical Load : Subsystem  Variant=on  VariantControlMode=label  LabelModeActiveChoice=1
  Wheel Angles : Subsystem
  FrntAxlF : Outport  Unit=N  VectorParamsAs1DForOutWhenUnconnected=off
  RearAxlF : Outport  Port=2  Unit=N  VectorParamsAs1DForOutWhenUnconnected=off
  Wheels : Outport  Port=3  VectorParamsAs1DForOutWhenUnconnected=off
  wires:
  Wheel Angles/1(WhlAngB) -> Veh2Tire/5(WhlAng)
  Constant/1 -> Tires/7(TirePrs)
  Constant3/1 -> Wheel Angles/2(camber), Tires/6(Camber)
  Veh2Tire/1(T) -> Tires/1(AxlTrq)
  Veh2Tire/2(P) -> Tires/2(BrkPrs)
  BrkPrs/1 -> Veh2Tire/2(BrkPrs)
  Veh2Tire/6(zdotAxle) -> Terminator2/1
  Veh2Tire/5(psidot) -> Tires/5(r)
  Velocity and Vertical Load/2(Fz) -> Tires/8(Fz)
  Velocity and Vertical Load/1(VehVel) -> Veh2Tire/4(VehVel)
  Axle Forces/1(FrntAxlF) -> FrntAxlF/1
  Axle Forces/2(RearAxlF) -> RearAxlF/1
  Tires/1(Wheel) -> Axle Forces/1(Wheel)
  Axle Forces/3(Wheels) -> Wheels/1
  VehFdbk/1 -> Axle Forces/2(VehFdbk), Bus Selector5/1, Velocity and Vertical Load/1(VehFdbk)
  Ground/1 -> Tires/10(Ground)
  WhlAng/1 -> Wheel Angles/1(steer)
  AxlTrq/1 -> Veh2Tire/1(AxlTrq)
  Friction/1 -> Tires/9(Friction)
  Bus Selector5/1 -> Veh2Tire/3(r)  "<r>"
  Veh2Tire/4(ydotAxle) -> Tires/4(Vy)
  Veh2Tire/3(xdotAxle) -> Tires/3(Vx)

== system vehicle_dynamics_blockset_simulation/Vehicle/Vehicle/Vehicle Body 3DOF External Longitudinal Wheels ==
  WhlAng : Inport
  "FwF " : Inport  Port=2
  "FwR " : Inport  Port=3
  WindXYZ : Inport  Port=4
  Bicycle : Subsystem  VariantControl=0
  Dual : Subsystem  VariantControl=1
  " Info" : Outport  VectorParamsAs1DForOutWhenUnconnected=off

== system vehicle_dynamics_blockset_simulation/Vehicle/Vehicle/Vehicle Signal Routing ==
  Info : Inport
  Ground : Inport  Port=2
  Bus Assignment : BusAssignment  AssignedSignals=InertFrm.Cg.Ang.phi,InertFrm.Cg.Ang.theta,InertFrm.Cg.Ang.psi,InertFrm.Geom.Disp.X,InertFrm.Geom.Disp.Y,InertFrm.Geom.Disp.Z
  Bus Selector4 : BusSelector  OutputSignals=InertFrm.Cg.Ang.phi,InertFrm.Cg.Ang.theta,InertFrm.Cg.Ang.psi  OutputAsBus=on
  Bus Selector6 : BusSelector  OutputSignals=InertFrm.Geom.Disp.X,InertFrm.Geom.Disp.Y,InertFrm.Geom.Disp.Z  OutputAsBus=on
  Bus to Vector3 : BusToVector
  Bus to Vector5 : BusToVector
  Demux : Demux  Outputs=3
  Demux1 : Demux  Outputs=3
  For 3D Visualization : MATLAB Function  TreatAsAtomicUnit=on  mask{trackW=VEHICLE.TRACK_FRONT, wheelB=VEHICLE.WHEEL_BASE}
      mask prompts: trackW "Vehicle track width, trackW [m]:"; wheelB "Vehicle wheelbase, wheelB [m]:"
      mask help: This block converts wheel ground height information into estimates of vehicle pitch, roll angles and vertical height in order to help in the visualization 3DOF based simulations with changes in terrain. Note that the resulting signals are only used as a visualization aid and do not account for the physical affects of the vehicle interacting with variable terrain or changes in orientation.
  Signal Specification : SignalSpecification  Unit=rad
  Signal Specification1 : SignalSpecification  Unit=rad
  Signal Specification2 : SignalSpecification  Unit=rad
  Signal Specification3 : SignalSpecification  Unit=m
  Signal Specification4 : SignalSpecification  Unit=m
  Signal Specification5 : SignalSpecification  Unit=m
  Veh : Outport  VectorParamsAs1DForOutWhenUnconnected=off
  wires:
  Info/1 -> Bus Selector4/1, Bus Selector6/1, Bus Assignment/1
  Bus to Vector3/1 -> For 3D Visualization/1(angleIn)
  For 3D Visualization/1(angles) -> Demux/1
  Bus Selector6/1 -> Bus to Vector5/1
  Ground/1 -> For 3D Visualization/3(Ground)
  For 3D Visualization/2(GeomXYZ) -> Demux1/1
  Bus to Vector5/1 -> For 3D Visualization/2(GemoXYZIn)
  Bus Selector4/1 -> Bus to Vector3/1
  Demux/2 -> Signal Specification1/1
  Demux/1 -> Signal Specification/1
  Demux/3 -> Signal Specification2/1
  Demux1/1 -> Signal Specification3/1
  Demux1/2 -> Signal Specification4/1
  Demux1/3 -> Signal Specification5/1
  Bus Assignment/1 -> Veh/1  "Veh"
  Signal Specification/1 -> Bus Assignment/2
  Signal Specification1/1 -> Bus Assignment/3
  Signal Specification2/1 -> Bus Assignment/4
  Signal Specification3/1 -> Bus Assignment/5
  Signal Specification4/1 -> Bus Assignment/6
  Signal Specification5/1 -> Bus Assignment/7

== system vehicle_dynamics_blockset_simulation/Vehicle/Wheels and tires/Axle Forces ==
  note: 1) Add Subsystem or Model blocks as valid variant choices.
      | 2) You cannot connect blocks at this level. At simulation, connectivity is automatically
      | determined, based on the active variant and port name matching.
  Wheel : Inport
  VehFdbk : Inport  Port=2
  Bicycle : Subsystem  VariantControl=0
  Dual : Subsystem  VariantControl=1
  FrntAxlF : Outport  Unit=N  VectorParamsAs1DForOutWhenUnconnected=off
  RearAxlF : Outport  Port=2  Unit=N  VectorParamsAs1DForOutWhenUnconnected=off
  Wheels : Outport  Port=3

== system vehicle_dynamics_blockset_simulation/Vehicle/Wheels and tires/Tire2Veh ==
  Wheels : Inport
  Bus Selector7 : BusSelector  OutputSignals=omega,Fx,Re,z,zdot,Kappa,Alpha
  Dead Zone2 : DeadZone  LowerValue=-5  UpperValue=5  ZeroCross=off  SaturateOnIntegerOverflow=on
  Demux : Demux  Outputs=[2,2]
  FwF : Outport  VectorParamsAs1DForOutWhenUnconnected=off
  FwR : Outport  Port=2  VectorParamsAs1DForOutWhenUnconnected=off
  omega : Outport  Port=3  VectorParamsAs1DForOutWhenUnconnected=off
  wires:
  Bus Selector7/2 -> Dead Zone2/1  "<Fx>"
  Dead Zone2/1 -> Demux/1  "Fx"
  Demux/1 -> FwF/1
  Wheels/1 -> Bus Selector7/1
  Bus Selector7/1 -> omega/1  "<omega>"
  Demux/2 -> FwR/1
